simulink model "Plant_C2"  (R2023a)
settings: Solver=ode45  StartTime=0.0  StopTime=200  RelTol=1e-2  EnableMultiTasking=on
values from neighbouring files (symbols this model uses):
  alfa = [alfaa alfab alfac alfad alfae alfaf]    [ChemBenchData.m]    (also in dati.m)
  H2 = [Hr2;He2*ones(Ne2,1);Hf2;Ha2*ones(Na2,1);Hc2]    [ChemBenchData.m]    (also in dati.m)
  N2 = Na2+Ne2+3    (= 19)    [ChemBenchData.m]    (also in dati.m = 9)
  Na2 = 8    [ChemBenchData.m]    (also in dati.m = 3)
  Ne2 = 8    [ChemBenchData.m]    (also in dati.m = 3)
  V2 = 385    [ChemBenchData.m]    (also in dati.m = 405)
  x2a = zeros(N2,1)    [ChemBenchData.m]    (also in dati.m)
  x2b = zeros(N2,1)    [ChemBenchData.m]    (also in dati.m)
  x2c = zeros(N2,1)    [ChemBenchData.m]    (also in dati.m)
undefined symbols (not defined in the file or in its folder): colonna2, somma, xk0_mod
settings Model: Creator=scattolini  LastModifiedBy=laura
settings SolverCC: AlgebraicLoopSolver=TrustRegion
settings DataIOCC: LimitDataPoints=on  SaveFormat=Array  SignalLoggingSaveFormat=ModelDataLogs  ReturnWorkspaceOutputs=off
settings OptimizationCC: BlockReduction=off  DefaultParameterBehavior=Inlined  InlineInvariantSignals=on  BufferReuse=off  ExpressionDepthLimit=2147483647  InitFltsAndDblsToZero=on  LifeSpan=inf
settings DebuggingCC: SaveWithParameterizedLinksMsg=none  UnderspecifiedInitializationDetection=Classic  MergeDetectMultiDrivingBlocksExec=none  SignalResolutionControl=TryResolveAllWithWarning  SolverPrmCheckMsg=warning  MultiTaskDSMMsg=warning  MultiTaskCondExecSysMsg=none  FcnCallInpInsideContextMsg=warning  UnconnectedInputMsg=warning  UnconnectedOutputMsg=warning  UnconnectedLineMsg=warning  StateNameClashWarn=warning  SFUnexpectedBacktrackingDiag=warning  SFNoUnconditionalDefaultTransitionDiag=warning  SFExecutionAtInitializationDiag=none  ArithmeticOperatorsInVariantConditions=warning
settings HardwareCC: ProdBitPerPointer=32  ProdBitPerSizeT=32  ProdBitPerPtrDiffT=32  ProdLargestAtomicFloat=None  ProdIntDivRoundTo=Undefined  ProdEndianess=Unspecified  ProdWordSize=32  ProdHWDeviceType=32-bit Generic
settings ModelReferenceCC: EnableRefExpFcnMdlSchedulingChecks=on  PropagateSignalLabelsOutOfModel=off
settings RTWCC: DLArmComputeVersion=19.05
settings CodeAppCC: StateflowObjectComments=on
settings GRTTargetCC: TargetFcnLib=ansi_tfl_tmw.mat  TargetLangStandard=C89/C90 (ANSI)  CombineOutputUpdateFcns=off  GRTInterface=on
settings ConfigComp: CovMetricSettings=dw  CovSaveCumulativeToWorkspaceVar=on  CovSaveSingleToWorkspaceVar=on

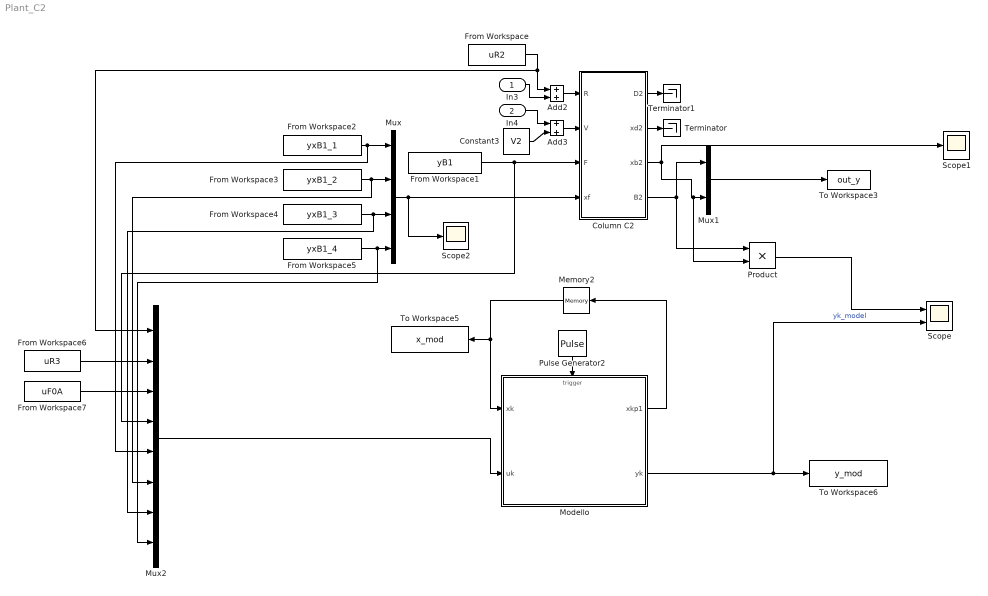
== system Plant_C2 ==
  In3 : Inport
  In4 : Inport  Port=2
  Add2 : Sum
  Add3 : Sum
  Column C2 : Subsystem
  Constant3 : Constant  Value=V2
  From Workspace : FromWorkspace  VariableName=uR2  SampleTime=-1
  From Workspace1 : FromWorkspace  VariableName=yB1  SampleTime=-1
  From Workspace2 : FromWorkspace  VariableName=yxB1_1  SampleTime=-1
  From Workspace3 : FromWorkspace  VariableName=yxB1_2  SampleTime=-1
  From Workspace4 : FromWorkspace  VariableName=yxB1_3  SampleTime=-1
  From Workspace5 : FromWorkspace  VariableName=yxB1_4  SampleTime=-1
  From Workspace6 : FromWorkspace  VariableName=uR3  SampleTime=-1
  From Workspace7 : FromWorkspace  VariableName=uF0A  SampleTime=-1
  Memory2 : Memory  InitialCondition=xk0_mod
  "Modello " : Subsystem  TreatAsAtomicUnit=on
  Mux : Mux
  Mux1 : Mux  Inputs=2
  Mux2 : Mux  Inputs=8
  Product : Product
  Pulse Generator2 : DiscretePulseGenerator  PulseType=Time based  Period=1  PulseWidth=5
  Scope : Scope  NumInputPorts=2
  Scope1 : Scope
  Scope2 : Scope
  Terminator : Terminator
  Terminator1 : Terminator
  To Workspace3 : ToWorkspace  VariableName=out_y  SampleTime=1
  To Workspace5 : ToWorkspace  VariableName=x_mod  SampleTime=1
  To Workspace6 : ToWorkspace  VariableName=y_mod  SampleTime=1
  wires:
  Add2/1 -> Column C2/1(R)
  From Workspace/1 -> Mux2/1, Add2/1
  Add3/1 -> Column C2/2(V)
  Constant3/1 -> Add3/2
  In3/1 -> Add2/2
  In4/1 -> Add3/1
  Column C2/2(xd2) -> Terminator/1
  Column C2/1(D2) -> Terminator1/1
  Mux1/1 -> To Workspace3/1
  From Workspace1/1 -> Mux2/4, Column C2/3(F)
  Mux/1 -> Scope2/1, Column C2/4(xf)
  From Workspace2/1 -> Mux2/5, Mux/1
  From Workspace4/1 -> Mux2/7, Mux/3
  From Workspace5/1 -> Mux2/8, Mux/4
  From Workspace3/1 -> Mux2/6, Mux/2
  Column C2/4(B2) -> Product/1, Mux1/1
  Column C2/3(xb2) -> Product/2, Mux1/2, Scope1/1
  "Modello "/1(xkp1) -> Memory2/1
  Memory2/1 -> "Modello "/1(xk), To Workspace5/1
  "Modello "/2(yk) -> Scope/2, To Workspace6/1  "yk_model"
  Pulse Generator2/1 -> "Modello "/Trigger
  Mux2/1 -> "Modello "/2(uk)
  From Workspace6/1 -> Mux2/2
  From Workspace7/1 -> Mux2/3
  Product/1 -> Scope/1

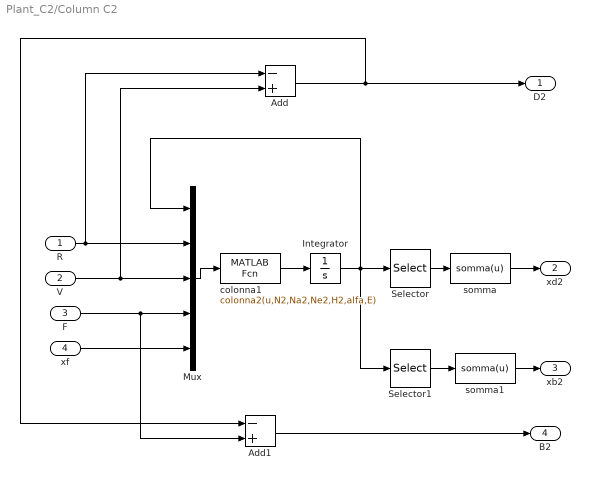
== system Plant_C2/Column C2 ==
  R : Inport
  V : Inport  Port=2
  F : Inport  Port=3
  xf : Inport  Port=4
  Add : Sum  Inputs=-+
  Add1 : Sum  Inputs=-+
  Integrator : Integrator  InitialCondition=[x2a;x2b;x2c]
  Mux : Mux  Inputs=5
  Selector : Selector  InputPortWidth=N2*3  IndexOptions=Index vector (dialog)  Indices=[N2 2*N2 3*N2]  OutputSizes=1
  Selector1 : Selector  InputPortWidth=N2*3  IndexOptions=Index vector (dialog)  Indices=[1 N2+1 2*N2+1]  OutputSizes=1
  colonna1 : MATLABFcn  MATLABFcn=colonna2(u,N2,Na2,Ne2,H2,alfa,E)  OutputDimensions=N2*3
  somma : MATLABFcn  MATLABFcn=somma(u)  OutputDimensions=4
  somma1 : MATLABFcn  MATLABFcn=somma(u)  OutputDimensions=4
  D2 : Outport
  xd2 : Outport  Port=2
  xb2 : Outport  Port=3
  B2 : Outport  Port=4
  wires:
  Mux/1 -> colonna1/1
  colonna1/1 -> Integrator/1
  Integrator/1 -> Selector/1, Mux/1, Selector1/1
  R/1 -> Mux/2, Add/1
  V/1 -> Mux/3, Add/2
  F/1 -> Mux/4, Add1/2
  xf/1 -> Mux/5
  Selector/1 -> somma/1
  somma/1 -> xd2/1
  Selector1/1 -> somma1/1
  somma1/1 -> xb2/1
  Add/1 -> D2/1, Add1/1
  Add1/1 -> B2/1

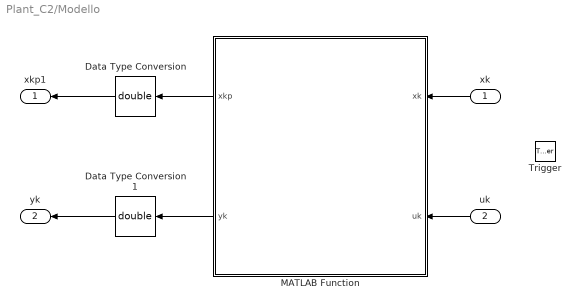
== system Plant_C2/Modello  ==
  xk : Inport
  uk : Inport  Port=2
  Trigger : TriggerPort  VariantControl=(inherit)
  Data Type Conversion : DataTypeConversion  OutDataTypeStr=double  RndMeth=Nearest  SaturateOnIntegerOverflow=off
  Data Type Conversion1 : DataTypeConversion  OutDataTypeStr=double  RndMeth=Nearest  SaturateOnIntegerOverflow=off
  MATLAB Function : MATLAB Function  TreatAsAtomicUnit=on
  xkp1 : Outport
  yk : Outport  Port=2
  wires:
  xk/1 -> MATLAB Function/1(xk)
  MATLAB Function/2(yk) -> Data Type Conversion1/1
  MATLAB Function/1(xkp) -> Data Type Conversion/1
  Data Type Conversion/1 -> xkp1/1
  Data Type Conversion1/1 -> yk/1
  uk/1 -> MATLAB Function/2(uk)

== matlab function Plant_C2/Modello /MATLAB Function ==
  data: xkp output; xk input; uk input; yk output
function [xkp, yk] = RNN(xk, uk)

    n_states = [3,3,3,3,3,3];
    layers_file = load("layers_file.mat");
    layers_file = layers_file.layers_file;
    input_scaler_bias = load("input_scaler_bias.mat");
    input_scaler_scale_common = load("input_scaler_scale_common.mat");
    output_scaler_bias = load("output_scaler_bias.mat");
    output_scaler_scale_common = load("output_scaler_scale_common.mat");

    % Scale input and output
    uk3_1 = (uk(1:3)  - (input_scaler_bias.input_scaler_bias(2:4)).') ./ (input_scaler_scale_common.input_scaler_scale_common).';
    uk3_2 = [uk(4)*uk(5); uk(4)*uk(6); uk(4)*uk(7); uk(4)*uk(8)];
    uk3_2 = (uk3_2  - (output_scaler_bias.output_scaler_bias(9:12)).') ./ (output_scaler_scale_common.output_scaler_scale_common).';

     
    % GRU 3
    uk3 = [uk3_1; uk3_2];
    xk3 = xk;
    zk3 = sigmoidfunction((layers_file.layers{1,5}.weights.Wzf(:,1:n_states(3))).' * uk3 + (layers_file.layers{1,5}.weights.Uzf(:,1:n_states(3))).' * xk3 + (layers_file.layers{1,5}.weights.bzf(:,1:n_states(3))).');
    fk3 = sigmoidfunction((layers_file.layers{1,5}.weights.Wzf(:,n_states(3)+1:end)).' * uk3 + (layers_file.layers{1,5}.weights.Uzf(:,n_states(3)+1:end)).' * xk3 + (layers_file.layers{1,5}.weights.bzf(:,n_states(3)+1:end)).');
    phi3 = tanh((layers_file.layers{1,5}.weights.Wr).' * uk3 + (layers_file.layers{1,5}.weights.Ur).' * (fk3.* xk3) + (layers_file.layers{1,5}.weights.br).');
    xkp3 = zk3 .* xk3 + (1-zk3) .* phi3;
    yk3 = layers_file.layers{1,6}.weights.weight * xk3 + (layers_file.layers{1,6}.weights.bias).';

    % Overall
    xkp = xkp3;
    yk = yk3;
    yk = yk .* (output_scaler_scale_common.output_scaler_scale_common).' + (output_scaler_bias.output_scaler_bias(13:16)).';
end
